simulink model "goodwin_linmod"  (R2024b)
settings: Solver=VariableStepAuto  StartTime=0.0  StopTime=tmax  MaxStep=1e-3
undefined symbols (not defined in the file or in its folder): alpha, beta, delta, nu, phi0, phi1, x10, x20
settings DataIOCC: ReturnWorkspaceOutputs=off

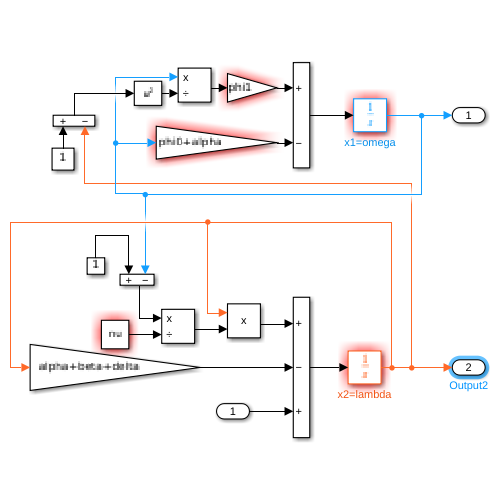
[thumbnail: Simulink's stored preview of the top-level diagram]
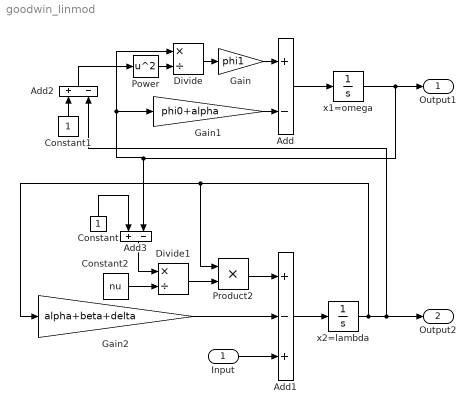
== system goodwin_linmod ==
  Input : Inport
  Add : Sum  Inputs=+-
  Add1 : Sum  Inputs=+-+
  Add2 : Sum  Inputs=+-
  Add3 : Sum  Inputs=+-
  Constant : Constant
  Constant1 : Constant
  Constant2 : Constant  Value=nu
  Divide : Product  Inputs=*/
  Divide1 : Product  Inputs=*/
  Gain : Gain  Gain=phi1
  Gain1 : Gain  Gain=phi0+alpha
  Gain2 : Gain  Gain=alpha+beta+delta
  Power : Math  Operator=square
  Product2 : Product
  x1=omega : Integrator  InitialCondition=x10
  x2=lambda : Integrator  InitialCondition=x20
  Output1 : Outport
  Output2 : Outport  Port=2
  wires:
  Product2/1 -> Add1/1
  Constant2/1 -> Divide1/2
  x2=lambda/1 -> Output2/1, Add2/2, Gain2/1, Product2/1
  Constant/1 -> Add3/1
  Power/1 -> Divide/2
  Gain2/1 -> Add1/2
  Constant1/1 -> Add2/1
  Gain1/1 -> Add/2
  Input/1 -> Add1/3
  Add3/1 -> Divide1/1
  Divide1/1 -> Product2/2
  Add2/1 -> Power/1
  x1=omega/1 -> Gain1/1, Divide/1, Add3/2, Output1/1
  Divide/1 -> Gain/1
  Add/1 -> x1=omega/1
  Add1/1 -> x2=lambda/1
  Gain/1 -> Add/1
